simulink model "assign3"  (Simulink 7.4)
settings: Solver=ode23  StartTime=0.0  StopTime=180  RelTol=1e-3
settings Model: Creator=Owner  LastModifiedBy=Owner

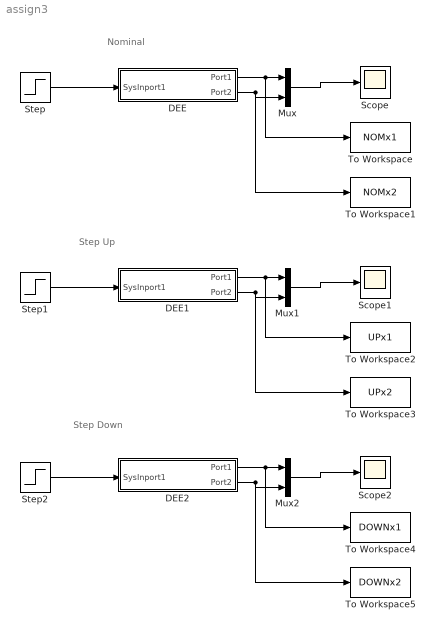
== system assign3 ==
  note: Nominal
  note: Step Up
  note: Step Down
  DEE : Subsystem
      settings: OpenFcn=diffeqed
      mask Type: Differential Equation Editor (DEE)
      mask Display: disp('Process Control')
  DEE1 : Subsystem
      settings: OpenFcn=diffeqed
      mask Type: Differential Equation Editor (DEE)
      mask Display: disp('Process Control')
  DEE2 : Subsystem
      settings: OpenFcn=diffeqed
      mask Type: Differential Equation Editor (DEE)
      mask Display: disp('Process Control')
  Mux : Mux  Inputs=2
  Mux1 : Mux  Inputs=2
  Mux2 : Mux  Inputs=2
  Scope : Scope
      settings: TimeRange=750
  Scope1 : Scope
  Scope2 : Scope
      settings: SaveName=ScopeData2
  Step : Step  Time=0  Before=3.5  After=3.5  SampleTime=0
  Step1 : Step  Time=0  Before=3.5  After=4  SampleTime=0
  Step2 : Step  Time=0  Before=3.5  After=3  SampleTime=0
  To Workspace : ToWorkspace  VariableName=NOMx1  SampleTime=-1  SaveFormat=Structure
  To Workspace1 : ToWorkspace  VariableName=NOMx2  SampleTime=-1  SaveFormat=Structure
  To Workspace2 : ToWorkspace  VariableName=UPx1  SampleTime=-1  SaveFormat=Structure
  To Workspace3 : ToWorkspace  VariableName=UPx2  SampleTime=-1  SaveFormat=Structure
  To Workspace4 : ToWorkspace  VariableName=DOWNx1  SampleTime=-1  SaveFormat=Structure
  To Workspace5 : ToWorkspace  VariableName=DOWNx2  SampleTime=-1  SaveFormat=Structure
  wires:
  DEE/1(Port1) -> Mux/1, To Workspace/1
  DEE/2(Port2) -> Mux/2, To Workspace1/1
  Mux/1 -> Scope/1
  Step/1 -> DEE/1(SysInport1)
  DEE1/1(Port1) -> Mux1/1, To Workspace2/1
  DEE1/2(Port2) -> Mux1/2, To Workspace3/1
  Mux1/1 -> Scope1/1
  Step1/1 -> DEE1/1(SysInport1)
  DEE2/1(Port1) -> Mux2/1, To Workspace4/1
  DEE2/2(Port2) -> Mux2/2, To Workspace5/1
  Mux2/1 -> Scope2/1
  Step2/1 -> DEE2/1(SysInport1)

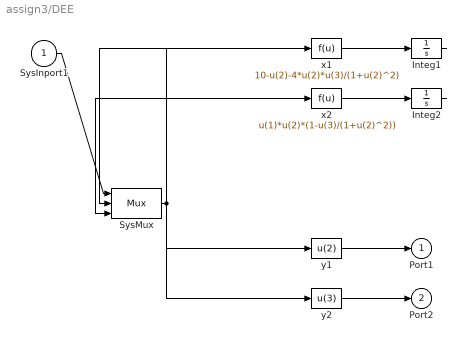
== system assign3/DEE ==
  SysInport1 : Inport
  Integ1 : Integrator
  Integ2 : Integrator  InitialCondition=2
  SysMux : Mux  Inputs=3
  x1 : Fcn  Expr=10-u(2)-4*u(2)*u(3)/(1+u(2)^2)
  x2 : Fcn  Expr=u(1)*u(2)*(1-u(3)/(1+u(2)^2))
  y1 : Fcn  Expr=u(2)
  y2 : Fcn  Expr=u(3)
  Port1 : Outport
  Port2 : Outport  Port=2
  wires:
  SysInport1/1 -> SysMux/1
  SysMux/1 -> x1/1, x2/1, y1/1, y2/1
  x1/1 -> Integ1/1
  Integ1/1 -> SysMux/2
  x2/1 -> Integ2/1
  Integ2/1 -> SysMux/3
  y1/1 -> Port1/1
  y2/1 -> Port2/1

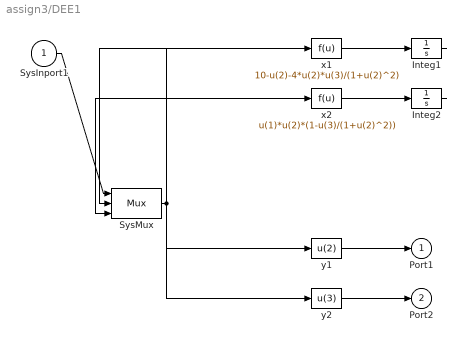
== system assign3/DEE1 ==
  SysInport1 : Inport
  Integ1 : Integrator
  Integ2 : Integrator  InitialCondition=2
  SysMux : Mux  Inputs=3
  x1 : Fcn  Expr=10-u(2)-4*u(2)*u(3)/(1+u(2)^2)
  x2 : Fcn  Expr=u(1)*u(2)*(1-u(3)/(1+u(2)^2))
  y1 : Fcn  Expr=u(2)
  y2 : Fcn  Expr=u(3)
  Port1 : Outport
  Port2 : Outport  Port=2
  wires:
  SysInport1/1 -> SysMux/1
  SysMux/1 -> x1/1, x2/1, y1/1, y2/1
  x1/1 -> Integ1/1
  Integ1/1 -> SysMux/2
  x2/1 -> Integ2/1
  Integ2/1 -> SysMux/3
  y1/1 -> Port1/1
  y2/1 -> Port2/1

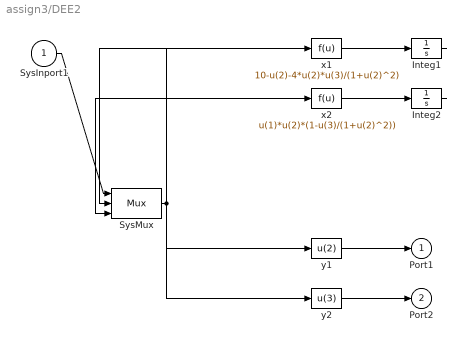
== system assign3/DEE2 ==
  SysInport1 : Inport
  Integ1 : Integrator
  Integ2 : Integrator  InitialCondition=2
  SysMux : Mux  Inputs=3
  x1 : Fcn  Expr=10-u(2)-4*u(2)*u(3)/(1+u(2)^2)
  x2 : Fcn  Expr=u(1)*u(2)*(1-u(3)/(1+u(2)^2))
  y1 : Fcn  Expr=u(2)
  y2 : Fcn  Expr=u(3)
  Port1 : Outport
  Port2 : Outport  Port=2
  wires:
  SysInport1/1 -> SysMux/1
  SysMux/1 -> x1/1, x2/1, y1/1, y2/1
  x1/1 -> Integ1/1
  Integ1/1 -> SysMux/2
  x2/1 -> Integ2/1
  Integ2/1 -> SysMux/3
  y1/1 -> Port1/1
  y2/1 -> Port2/1
